simulink model "TVCrocketSim_6DOF_MAIN"  (R2022b)
settings: Solver=VariableStepAuto  StartTime=0.0  StopTime=MAX_SIM_TIME  FixedStep=dt  RelTol=1e-6
InitFcn:
  | TVCrocketSim_6DOF_INIT
StopFcn:
  | TVCrocketSim_6DOF_POST
values from neighbouring files (symbols this model uses):
  CTRL_ON = 1    [TVCrocketSim_6DOF_INIT.m]
  GUIDANCE_ON = 1    [TVCrocketSim_6DOF_INIT.m]
libraries: slpidlib x1
settings Model: Creator=c09wy  LastModifiedBy=c09wy
settings SolverCC: AlgebraicLoopSolver=TrustRegion
settings DataIOCC: ReturnWorkspaceOutputs=off
settings DebuggingCC: UnconnectedInputMsg=warning  UnconnectedOutputMsg=warning  UnconnectedLineMsg=warning  SFMachineParentedDataDiag=warning  UnderSpecifiedDimensionMsg=warning  ArithmeticOperatorsInVariantConditions=warning
settings ModelReferenceCC: EnableRefExpFcnMdlSchedulingChecks=on
settings SFSimCC: CustomCodeUndefinedFunction=UseInterfaceOnly

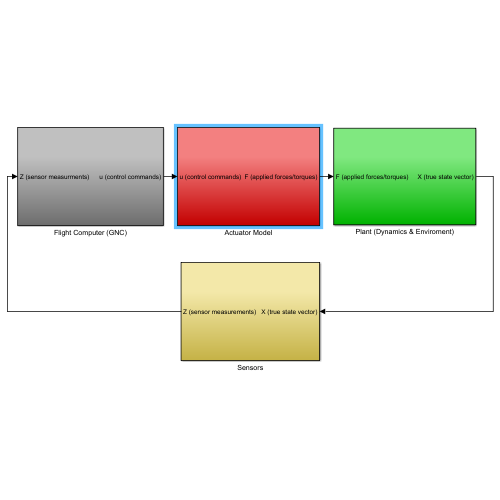
[thumbnail: Simulink's stored preview of the top-level diagram]
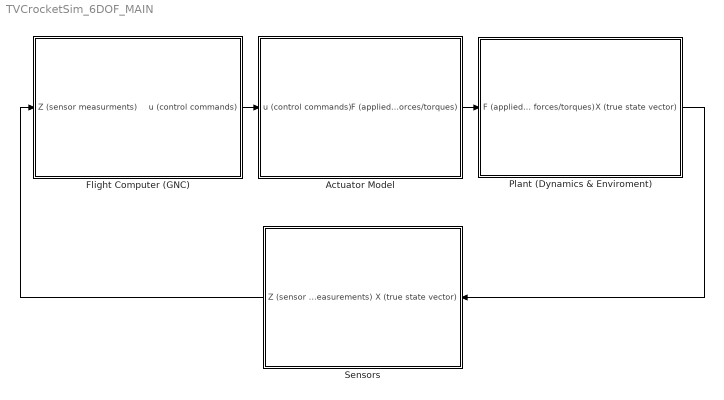
== system TVCrocketSim_6DOF_MAIN ==
  Actuator Model : Subsystem
  Flight Computer (GNC) : Subsystem
  Plant (Dynamics & Enviroment) : Subsystem
  Sensors : Subsystem
  wires:
  Plant (Dynamics & Enviroment)/1(X (true state vector)) -> Sensors/1(X (true state vector))
  Actuator Model/1(F (applied forces/torques)) -> Plant (Dynamics & Enviroment)/1(F (applied forces/torques))
  Sensors/1(Z (sensor measurements)) -> Flight Computer (GNC)/1(Z (sensor measurments))
  Flight Computer (GNC)/1(u (control commands)) -> Actuator Model/1(u (control commands))

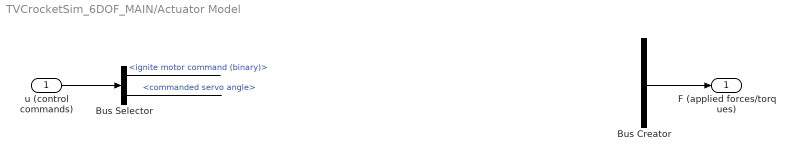
== system TVCrocketSim_6DOF_MAIN/Actuator Model ==
  u (control commands) : Inport
  Bus Creator : BusCreator  Inputs=2
  Bus Selector : BusSelector  OutputSignals=ignite motor command (binary),commanded servo angle
  F (applied forces/torques) : Outport  VectorParamsAs1DForOutWhenUnconnected=off
  wires:
  Bus Creator/1 -> F (applied forces/torques)/1
  ? -> Bus Creator/1  "F_thrust (motor thrust vector)"
  u (control commands)/1 -> Bus Selector/1
  Bus Selector/1 -> ?  "<ignite motor command (binary)>"
  Bus Selector/2 -> ?  "<commanded servo angle>"
  ? -> Bus Creator/2  "Tau_thrust (Torque applied by rocket motor about body CoM)"

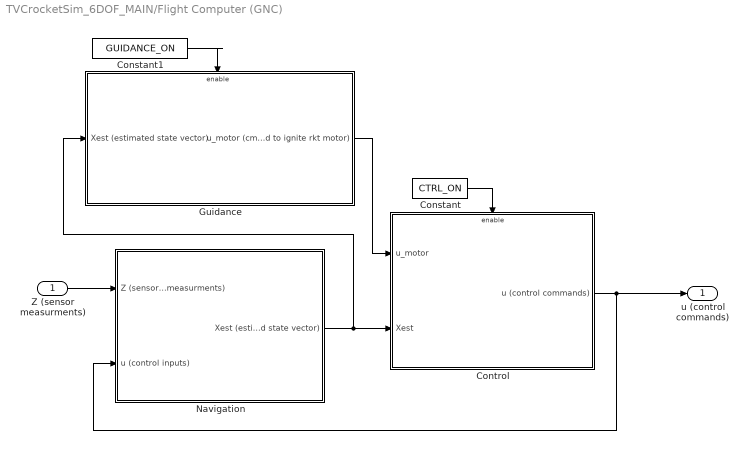
== system TVCrocketSim_6DOF_MAIN/Flight Computer (GNC) ==
  Z (sensor measurments) : Inport
  Constant : Constant  Value=CTRL_ON
  Constant1 : Constant  Value=GUIDANCE_ON
  Control : Subsystem
  Guidance : Subsystem
  Navigation : Subsystem
  u (control commands) : Outport  VectorParamsAs1DForOutWhenUnconnected=off
  wires:
  Constant/1 -> Control/Enable
  Z (sensor measurments)/1 -> Navigation/1(Z (sensor measurments))
  Constant1/1 -> Guidance/Enable
  Navigation/1(Xest (estimated state vector)) -> Guidance/1(Xest (estimated state vector)), Control/2("Xest ")
  Guidance/1(u_motor (cmd to ignite rkt motor)) -> Control/1(u_motor)
  Control/1(u (control commands)) -> u (control commands)/1, Navigation/2(u (control inputs))

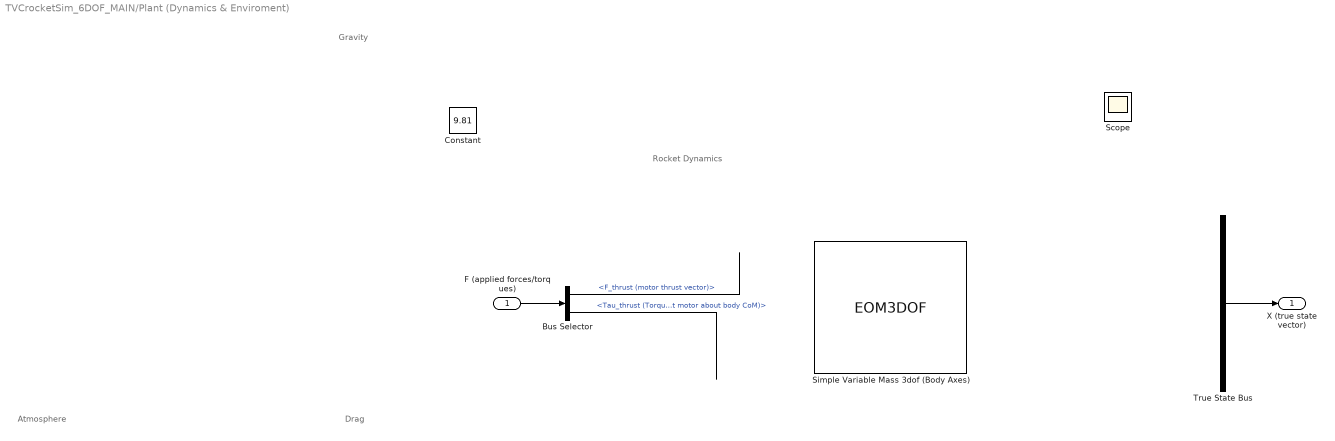
== system TVCrocketSim_6DOF_MAIN/Plant (Dynamics & Enviroment) ==
  note: Rocket Dynamics
  note: Gravity
  note: Atmosphere
  note: Drag
  F (applied forces/torques) : Inport
  Bus Selector : BusSelector  OutputSignals=F_thrust (motor thrust vector),Tau_thrust (Torque applied by rocket motor about body CoM)
  Constant : Constant  Value=9.81
  Scope : Scope
  Simple Variable Mass 3dof (Body Axes) : EOM3DOF  mtype=Simple Variable
  True State Bus : BusCreator  Inputs=5
  X (true state vector) : Outport  VectorParamsAs1DForOutWhenUnconnected=off
  wires:
  ? -> True State Bus/1  "x_n_nb (true postion in inertial frame)"
  ? -> True State Bus/2  "xDot_n_nb (true velocity in inertial frame)"
  ? -> True State Bus/3  "xDotDot_n_nb (true acceleration in navigation frame)"
  ? -> True State Bus/4  "q_n_b (quaternion of body WRT nav frame)"
  ? -> True State Bus/5  "w_n_bn (angular velocity of body WRT nav frame)"
  True State Bus/1 -> X (true state vector)/1
  F (applied forces/torques)/1 -> Bus Selector/1
  Bus Selector/1 -> ?  "<F_thrust (motor thrust vector)>"
  Bus Selector/2 -> ?  "<Tau_thrust (Torque applied by rocket motor about body CoM)>"
  ? -> Scope/1

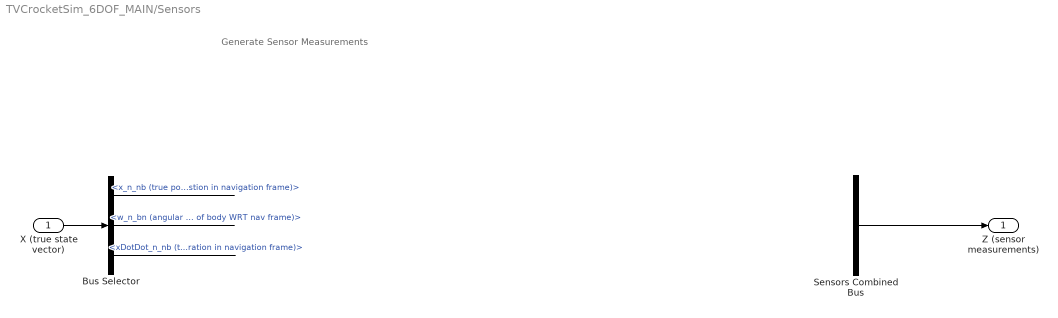
== system TVCrocketSim_6DOF_MAIN/Sensors ==
  note: Generate Sensor Measurements
  X (true state vector) : Inport
  Bus Selector : BusSelector  OutputSignals=x_n_nb (true postion in navigation frame),w_n_bn (angular velocity of body WRT nav frame),xDotDot_n_nb (true acceleration in navigation frame)
  Sensors Combined Bus : BusCreator  Inputs=3
  Z (sensor measurements) : Outport
  wires:
  ? -> Sensors Combined Bus/1  "Z_accelerometer (specific force measurement vector)"
  ? -> Sensors Combined Bus/2  "Z_gyroscope (angular velocity vector)"
  ? -> Sensors Combined Bus/3  "Z_baroAlt (pressure altitude from baro sensor)"
  Sensors Combined Bus/1 -> Z (sensor measurements)/1
  X (true state vector)/1 -> Bus Selector/1
  Bus Selector/1 -> ?  "<x_n_nb (true postion in navigation frame)>"
  Bus Selector/2 -> ?  "<w_n_bn (angular velocity of body WRT nav frame)>"
  Bus Selector/3 -> ?  "<xDotDot_n_nb (true acceleration in navigation frame)>"

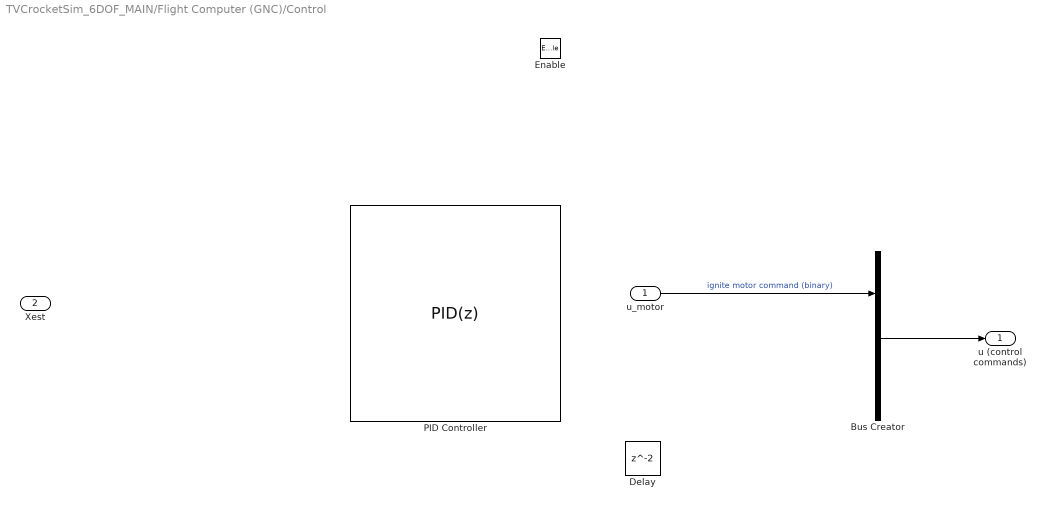
== system TVCrocketSim_6DOF_MAIN/Flight Computer (GNC)/Control ==
  u_motor : Inport
  "Xest " : Inport  Port=2
  Enable : EnablePort
  Bus Creator : BusCreator  Inputs=2
  Delay : Delay  SampleTime=.01
  PID Controller : slpidlib/PID Controller  Controller=PID  Form=Parallel  TimeDomain=Discrete-time  UseExternalTs=off  SampleTime=.01  IntegratorMethod=Forward Euler  FilterMethod=Forward Euler  ControllerParametersSource=internal  P=1  I=1  UseKiTs=off  D=0  N=100  UseFilter=on  TunerSelectOption=Transfer Function Based (PID Tuner App)  InitialConditionSource=internal  InitialConditionForIntegrator=0  InitialConditionForFilter=0  DifferentiatorICPrevScaledInput=0  ExternalReset=none  TrackingMode=off  Kt=1  LimitOutput=off  SatLimitsSource=internal  UpperSaturationLimit=inf  LowerSaturationLimit=-inf  LinearizeAsGain=on  AntiWindupMode=none  Kb=1  LimitIntegrator=off  UpperIntegratorSaturationLimit=inf  LowerIntegratorSaturationLimit=-inf  POutMin=[]  POutMax=[]  IOutMin=[]  IOutMax=[]  DOutMin=[]  DOutMax=[]  NOutMin=[]  NOutMax=[]  SumOutMin=[]  SumOutMax=[]  SaturationOutMin=[]  SaturationOutMax=[]  PParamMin=[]  PParamMax=[]  IParamMin=[]  IParamMax=[]  DParamMin=[]  DParamMax=[]  NParamMin=[]  NParamMax=[]  KbParamMin=[]  KbParamMax=[]  KtParamMin=[]  KtParamMax=[]  KbOutMin=[]  KbOutMax=[]  KtOutMin=[]  KtOutMax=[]  IntegratorOutMin=[]  IntegratorOutMax=[]  FilterOutMin=[]  FilterOutMax=[]  SumI1OutMin=[]  SumI1OutMax=[]  SumI2OutMin=[]  SumI2OutMax=[]  SumI3OutMin=[]  SumI3OutMax=[]  SumI4OutMin=[]  SumI4OutMax=[]  SumDOutMin=[]  SumDOutMax=[]  DifferentiatorOutMin=[]  DifferentiatorOutMax=[]  FilterDiffOutCoefMin=[]  FilterDiffOutCoefMax=[]  ReciprocalOutMin=[]  ReciprocalOutMax=[]  SumDenOutMin=[]  SumDenOutMax=[]  SumNumOutMin=[]  SumNumOutMax=[]  DivideOutMin=[]  DivideOutMax=[]  UdiffTsProdOutMin=[]  UdiffTsProdOutMax=[]  NTsProdOutMin=[]  NTsProdOutMax=[]  UintegralTsProdOutMin=[]  UintegralTsProdOutMax=[]  UngainTsProdOutMin=[]  UngainTsProdOutMax=[]  ClampingZeroOutDataTypeStr=Inherit: Inherit via back propagation  ClampingZeroOutMin=[]  ClampingZeroOutMax=[]  FilterDenConstantOutDataTypeStr=Inherit: Inherit via back propagation  FilterDenConstantOutMin=[]  FilterDenConstantOutMax=[]  PCopyOutDataTypeStr=Inherit: Inherit via back propagation  PCopyOutMin=[]  PCopyOutMax=[]  NCopyOutDataTypeStr=Inherit: Inherit via back propagation  NCopyOutMin=[]  NCopyOutMax=[]  IntegratorContinuousStateAttributes=''  IntegratorStateMustResolveToSignalObject=off  IntegratorRTWStateStorageClass=Auto  FilterContinuousStateAttributes=''  FilterStateMustResolveToSignalObject=off  FilterRTWStateStorageClass=Auto  ParallelPVariant=InternalParameters  IdealPVariant=Disabled  IVariant=InternalParameters  DVariant=InternalParameters  IntegratorVariant=Discrete  SatVariant=Disabled  AWVariant=Passthrough  PCopyVariant=Disabled  TRVariant=Disabled  FdbkBlocksVariant=Forward  IdealPFdbkVariant=Disabled  SatFdbkVariant=Disabled  DerivativeFilterVariant=ForwardEulerFilter  NVariant=InternalParameters  NCopyVariant=Disabled  FilterICVariant=InternalICsFilter  IntegratorICVariant=InternalICs  ExternalResetVariant=Disabled  TRSumVariant=Passthrough  SumFdbkVariant=Disabled  SumVariant=Sum_PID  TsampFilterVariant=InternalTs  TsampNgainVariant=Passthrough  TsampIntegralVariant=Passthrough  ExternalSaturationOutDataTypeStr=Inherit: Same as second input
  u (control commands) : Outport
  wires:
  ? -> Bus Creator/2  "commanded servo angle"
  u_motor/1 -> Bus Creator/1  "ignite motor command (binary)"
  Bus Creator/1 -> u (control commands)/1

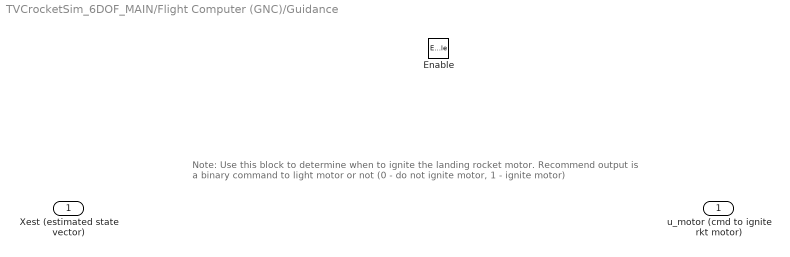
== system TVCrocketSim_6DOF_MAIN/Flight Computer (GNC)/Guidance ==
  note: Note: Use this block to determine when to ignite the landing rocket motor. Recommend output is a binary command to light motor or not (0 - do not ignite motor, 1 - ignite motor)
  Xest (estimated state vector) : Inport
  Enable : EnablePort
  u_motor (cmd to ignite rkt motor) : Outport  VectorParamsAs1DForOutWhenUnconnected=off

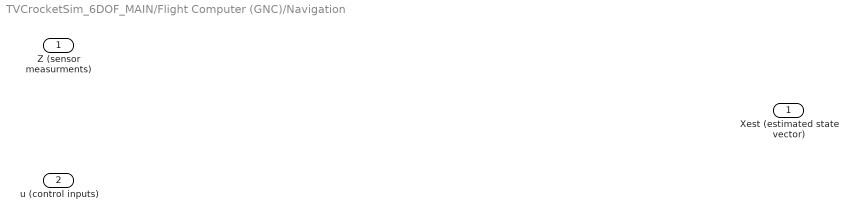
== system TVCrocketSim_6DOF_MAIN/Flight Computer (GNC)/Navigation ==
  Z (sensor measurments) : Inport
  u (control inputs) : Inport  Port=2
  Xest (estimated state vector) : Outport  VectorParamsAs1DForOutWhenUnconnected=off
